simulink model "SimpleHumidifier_std"  (R2023b)
settings: Solver=ode4  StartTime=0.0  StopTime=10.0  FixedStep=1e-4  RelTol=1e-6
undefined symbols (not defined in the file): p_in_dry, p_in_wet, RH_in_dry, RH_in_wet, T_in_dry, T_in_wet, W_in_dry, W_in_wet, yO2_in_dry, yO2_in_wet
libraries: slpidlib x1
settings Model: Creator=KOTA-Z  LastModifiedBy=KOTA-Z

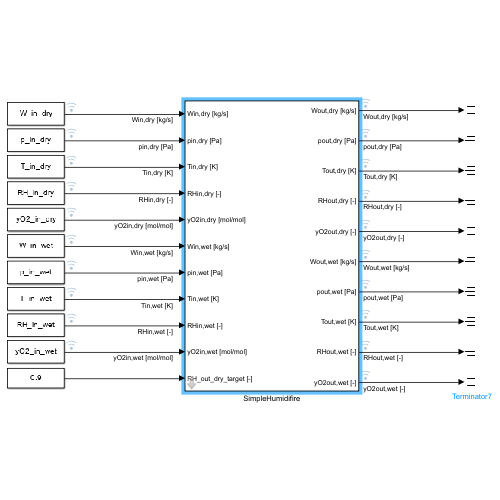
[thumbnail: Simulink's stored preview of the top-level diagram]
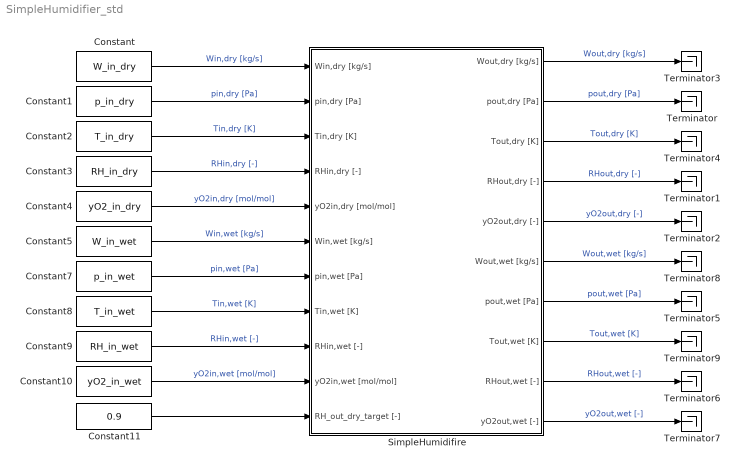
== system SimpleHumidifier_std ==
  Constant : Constant  Value=W_in_dry
  Constant1 : Constant  Value=p_in_dry
  Constant10 : Constant  Value=yO2_in_wet
  Constant11 : Constant  Value=0.9
  Constant2 : Constant  Value=T_in_dry
  Constant3 : Constant  Value=RH_in_dry
  Constant4 : Constant  Value=yO2_in_dry
  Constant5 : Constant  Value=W_in_wet
  Constant7 : Constant  Value=p_in_wet
  Constant8 : Constant  Value=T_in_wet
  Constant9 : Constant  Value=RH_in_wet
  SimpleHumidifire : Subsystem  mask(Simple FCstack){V_ca=1, A_ca=1, R_N2=1, R_O2=1, R_H2O=1, M_N2=1, M_O2=1, M_H2O=1}
      mask prompts: V_ca "Stack Volume (Cathode side) [m^3]"; A_ca "Stack Flow area (Cathode side) [m^2]"; R_N2 "Gas Constant N2 [J/kg/K]"; R_O2 "Gas Constant O2 [J/kg/K]"; R_H2O "Gas Constant H2O [J/kg/K]"; M_N2 "Molecular Weight N2 [kg/mol]"; M_O2 "Molecular Weight O2 [kg/mol]"; M_H2O "Molecular Weight H2O [kg/mol]"
      mask help: This block provides a simplified FCstack model. The reacted O2 and generated H2O in the stack are calculated based on lambda. Delay due to volume is considered and the pressure drop is approximated as the orifice law.
      mask DialogControl ParameterGroupVar Prompt: Geometric parameter
      mask DialogControl Container3 Prompt: Physical property
  Terminator{,1..9} (10 alike) : Terminator
  wires:
  Constant4/1 -> SimpleHumidifire/5(yO2in,dry [mol/mol])  "yO2in,dry [mol/mol]"
  Constant/1 -> SimpleHumidifire/1(Win,dry [kg/s])  "Win,dry [kg/s]"
  Constant3/1 -> SimpleHumidifire/4(RHin,dry [-])  "RHin,dry [-]"
  Constant1/1 -> SimpleHumidifire/2(pin,dry [Pa])  "pin,dry [Pa]"
  SimpleHumidifire/4(RHout,dry [-]) -> Terminator1/1  "RHout,dry [-]"
  SimpleHumidifire/1(Wout,dry [kg/s]) -> Terminator3/1  "Wout,dry [kg/s]"
  SimpleHumidifire/2(pout,dry [Pa]) -> Terminator/1  "pout,dry [Pa]"
  SimpleHumidifire/5(yO2out,dry [-]) -> Terminator2/1  "yO2out,dry [-]"
  Constant2/1 -> SimpleHumidifire/3(Tin,dry [K])  "Tin,dry [K]"
  SimpleHumidifire/3(Tout,dry [K]) -> Terminator4/1  "Tout,dry [K]"
  Constant8/1 -> SimpleHumidifire/8(Tin,wet [K])  "Tin,wet [K]"
  Constant5/1 -> SimpleHumidifire/6(Win,wet [kg/s])  "Win,wet [kg/s]"
  Constant7/1 -> SimpleHumidifire/7(pin,wet [Pa])  "pin,wet [Pa]"
  Constant9/1 -> SimpleHumidifire/9(RHin,wet [-])  "RHin,wet [-]"
  Constant10/1 -> SimpleHumidifire/10(yO2in,wet [mol/mol])  "yO2in,wet [mol/mol]"
  SimpleHumidifire/6(Wout,wet [kg/s]) -> Terminator8/1  "Wout,wet [kg/s]"
  SimpleHumidifire/10(yO2out,wet [-]) -> Terminator7/1  "yO2out,wet [-]"
  SimpleHumidifire/7(pout,wet [Pa]) -> Terminator5/1  "pout,wet [Pa]"
  SimpleHumidifire/9(RHout,wet [-]) -> Terminator6/1  "RHout,wet [-]"
  SimpleHumidifire/8(Tout,wet [K]) -> Terminator9/1  "Tout,wet [K]"
  Constant11/1 -> SimpleHumidifire/11(RH_out_dry_target [-])

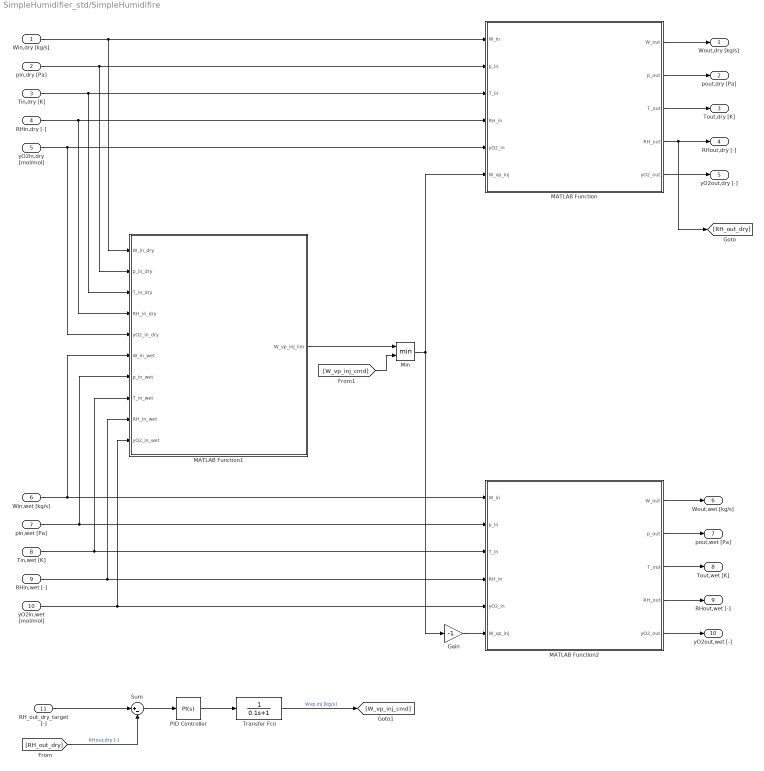
== system SimpleHumidifier_std/SimpleHumidifire ==
  Win,dry [kg/s] : Inport
  pin,dry [Pa] : Inport  Port=2
  Tin,dry [K] : Inport  Port=3
  RHin,dry [-] : Inport  Port=4
  yO2in,dry [mol/mol] : Inport  Port=5
  Win,wet [kg/s] : Inport  Port=6
  pin,wet [Pa] : Inport  Port=7
  Tin,wet [K] : Inport  Port=8
  RHin,wet [-] : Inport  Port=9
  yO2in,wet [mol/mol] : Inport  Port=10
  RH_out_dry_target [-] : Inport  Port=11
  Gain : Gain  Gain=-1
  MATLAB Function : MATLAB Function  TreatAsAtomicUnit=on
  MATLAB Function1 : MATLAB Function  TreatAsAtomicUnit=on
  MATLAB Function2 : MATLAB Function  TreatAsAtomicUnit=on
  Min : MinMax  Inputs=2
  PID Controller : slpidlib/PID Controller  Controller=PI  Form=Parallel  TimeDomain=Continuous-time  UseExternalTs=off  SampleTime=-1  IntegratorMethod=Forward Euler  FilterMethod=Forward Euler  ControllerParametersSource=internal  P=1  I=10  UseKiTs=off  D=0  N=100  UseFilter=on  TunerSelectOption=Transfer Function Based (PID Tuner App)  InitialConditionSource=internal  InitialConditionForIntegrator=0  InitialConditionForFilter=0  DifferentiatorICPrevScaledInput=0  ExternalReset=none  TrackingMode=off  Kt=1  LimitOutput=on  SatLimitsSource=internal  UpperSaturationLimit=1  LowerSaturationLimit=0  LinearizeAsGain=on  AntiWindupMode=back-calculation  Kb=1  LimitIntegrator=off  UpperIntegratorSaturationLimit=inf  LowerIntegratorSaturationLimit=-inf  POutMin=[]  POutMax=[]  IOutMin=[]  IOutMax=[]  DOutMin=[]  DOutMax=[]  NOutMin=[]  NOutMax=[]  SumOutMin=[]  SumOutMax=[]  SaturationOutMin=[]  SaturationOutMax=[]  PParamMin=[]  PParamMax=[]  IParamMin=[]  IParamMax=[]  DParamMin=[]  DParamMax=[]  NParamMin=[]  NParamMax=[]  KbParamMin=[]  KbParamMax=[]  KtParamMin=[]  KtParamMax=[]  KbOutMin=[]  KbOutMax=[]  KtOutMin=[]  KtOutMax=[]  IntegratorOutMin=[]  IntegratorOutMax=[]  FilterOutMin=[]  FilterOutMax=[]  SumI1OutMin=[]  SumI1OutMax=[]  SumI2OutMin=[]  SumI2OutMax=[]  SumI3OutMin=[]  SumI3OutMax=[]  SumI4OutMin=[]  SumI4OutMax=[]  SumDOutMin=[]  SumDOutMax=[]  DifferentiatorOutMin=[]  DifferentiatorOutMax=[]  FilterDiffOutCoefMin=[]  FilterDiffOutCoefMax=[]  ReciprocalOutMin=[]  ReciprocalOutMax=[]  SumDenOutMin=[]  SumDenOutMax=[]  SumNumOutMin=[]  SumNumOutMax=[]  DivideOutMin=[]  DivideOutMax=[]  UdiffTsProdOutMin=[]  UdiffTsProdOutMax=[]  NTsProdOutMin=[]  NTsProdOutMax=[]  UintegralTsProdOutMin=[]  UintegralTsProdOutMax=[]  UngainTsProdOutMin=[]  UngainTsProdOutMax=[]  ClampingZeroOutDataTypeStr=Inherit: Inherit via back propagation  ClampingZeroOutMin=[]  ClampingZeroOutMax=[]  FilterDenConstantOutDataTypeStr=Inherit: Inherit via back propagation  FilterDenConstantOutMin=[]  FilterDenConstantOutMax=[]  PCopyOutDataTypeStr=Inherit: Inherit via back propagation  PCopyOutMin=[]  PCopyOutMax=[]  NCopyOutDataTypeStr=Inherit: Inherit via back propagation  NCopyOutMin=[]  NCopyOutMax=[]  IntegratorContinuousStateAttributes=''  IntegratorStateMustResolveToSignalObject=off  IntegratorRTWStateStorageClass=Auto  FilterContinuousStateAttributes=''  FilterStateMustResolveToSignalObject=off  FilterRTWStateStorageClass=Auto  ParallelPVariant=InternalParameters  IdealPVariant=Disabled  IVariant=InternalParameters  DVariant=Disabled  IntegratorVariant=Continuous  SatVariant=Enabled  AWVariant=BackCalculation  PCopyVariant=Disabled  TRVariant=Disabled  FdbkBlocksVariant=Forward  IdealPFdbkVariant=Disabled  SatFdbkVariant=Disabled  DerivativeFilterVariant=Disabled  NVariant=Disabled  NCopyVariant=Disabled_SignalSpec  FilterICVariant=Disabled  IntegratorICVariant=InternalICs  ExternalResetVariant=Disabled  TRSumVariant=Passthrough  SumFdbkVariant=Disabled  SumVariant=Sum_PI  TsampFilterVariant=InternalTs  TsampNgainVariant=Passthrough  TsampIntegralVariant=Disabled_SignalSpec  ExternalSaturationOutDataTypeStr=Inherit: Same as second input
  Sum : Sum  Inputs=|+-
  Transfer Fcn : TransferFcn  Denominator=[0.1 1]
  Wout,dry [kg/s] : Outport
  pout,dry [Pa] : Outport  Port=2
  Tout,dry [K] : Outport  Port=3
  RHout,dry [-] : Outport  Port=4
  yO2out,dry [-] : Outport  Port=5
  Wout,wet [kg/s] : Outport  Port=6
  pout,wet [Pa] : Outport  Port=7
  Tout,wet [K] : Outport  Port=8
  RHout,wet [-] : Outport  Port=9
  yO2out,wet [-] : Outport  Port=10
  wires:
  MATLAB Function/5(yO2_out) -> yO2out,dry [-]/1
  MATLAB Function/2(p_out) -> pout,dry [Pa]/1
  MATLAB Function/1(W_out) -> Wout,dry [kg/s]/1
  MATLAB Function/4(RH_out) -> [RH_out_dry], RHout,dry [-]/1
  MATLAB Function/3(T_out) -> Tout,dry [K]/1
  pin,wet [Pa]/1 -> MATLAB Function1/7(p_in_wet), MATLAB Function2/2(p_in)
  Win,wet [kg/s]/1 -> MATLAB Function2/1(W_in), MATLAB Function1/6(W_in_wet)
  RHin,wet [-]/1 -> MATLAB Function1/9(RH_in_wet), MATLAB Function2/4(RH_in)
  RHin,dry [-]/1 -> MATLAB Function1/4(RH_in_dry), MATLAB Function/4(RH_in)
  pin,dry [Pa]/1 -> MATLAB Function1/2(p_in_dry), MATLAB Function/2(p_in)
  Tin,dry [K]/1 -> MATLAB Function1/3(T_in_dry), MATLAB Function/3(T_in)
  Win,dry [kg/s]/1 -> MATLAB Function1/1(W_in_dry), MATLAB Function/1(W_in)
  yO2in,wet [mol/mol]/1 -> MATLAB Function1/10(yO2_in_wet), MATLAB Function2/5(yO2_in)
  yO2in,dry [mol/mol]/1 -> MATLAB Function1/5(yO2_in_dry), MATLAB Function/5(yO2_in)
  Tin,wet [K]/1 -> MATLAB Function1/8(T_in_wet), MATLAB Function2/3(T_in)
  [W_vp_inj_cmd] -> Min/2
  MATLAB Function1/1(W_vp_inj_lim) -> Min/1
  Min/1 -> MATLAB Function/6(W_vp_inj), Gain/1
  Gain/1 -> MATLAB Function2/6(W_vp_inj)
  MATLAB Function2/1(W_out) -> Wout,wet [kg/s]/1
  MATLAB Function2/2(p_out) -> pout,wet [Pa]/1
  MATLAB Function2/3(T_out) -> Tout,wet [K]/1
  MATLAB Function2/4(RH_out) -> RHout,wet [-]/1
  MATLAB Function2/5(yO2_out) -> yO2out,wet [-]/1
  PID Controller/1 -> Transfer Fcn/1
  Transfer Fcn/1 -> [W_vp_inj_cmd]  "Wvp,inj [kg/s]"
  Sum/1 -> PID Controller/1
  RH_out_dry_target [-]/1 -> Sum/1
  [RH_out_dry] -> Sum/2  "RHout,dry [-]"

== matlab function SimpleHumidifier_std/SimpleHumidifire/MATLAB Function ==
  data: W_in input; W_out output; p_in input; T_in input; RH_in input; yO2_in input; W_vp_inj input; p_out output; T_out output; RH_out output; yO2_out output
%% 加湿／除湿計算（分圧ベース計算）
function [W_out, p_out, T_out, RH_out, yO2_out] = HM_std(W_in, p_in, T_in, RH_in, yO2_in, W_vp_inj)
    % 湿り空気の状態計算
    [W_O2_in, W_N2_in, W_vp_in, p_O2_in, p_N2_in, p_vp_in, M_in, R_in, cp_in, kap_in] = calc_MA_property(W_in, p_in, T_in, RH_in, yO2_in);

    % 水蒸気の注入
    W_vp_out = W_vp_in + W_vp_inj;  % [kg/s]

    % 出口流量計算
    W_O2_out = W_O2_in; % [kg/s]
    W_N2_out = W_N2_in; % [kg/s]
    W_out = W_O2_out + W_N2_out + W_vp_out; % [kg/s]

    % 出口圧計算
    p_O2_out = p_O2_in; % [Pa]
    p_N2_out = p_N2_in; % [Pa]
    if W_vp_out <= 0
        p_vp_out = 0;
    else
        p_vp_out = W_vp_out/W_vp_in * p_vp_in;  % [Pa]
    end
    p_out = p_O2_out + p_N2_out + p_vp_out;     % [Pa]

    % 温度は一定とする
    T_out = T_in;       % [K]

    % 相対湿度計算
    RH_out = p_vp_out/sat_vp_pressure(T_out);

    % 空気組成は一定とする
    yO2_out = yO2_in;   % [-]
end

%% 湿り空気の状態量計算
function [W_O2, W_N2, W_vp, p_O2, p_N2, p_vp, M, R, cp, kap] = calc_MA_property(W, p, T, RH, yO2)
    % 物理定数の定義
    % 分子量定義
    M_O2 = 32e-3;   % [kg/mol]
    M_N2 = 28e-3;   % [kg/mol]
    M_vp = 18e-3;   % [kg/mol]
    % 気体定数定義
    R0 = 8.31446261815324; % [J/K/mol]
    
    % 分圧計算
    p_vp_sat = sat_vp_pressure(T);
    p_vp = RH * p_vp_sat;
    p_DA = p - p_vp;
    p_O2 = yO2 * p_DA;
    p_N2 = p_DA - p_O2;
    
    % 湿り空気のモル分率計算
    x_O2 = p_O2/p;
    x_N2 = p_N2/p;
    x_vp = p_vp/p;

    % 湿り空気の分子量計算
    M = M_O2*x_O2 + M_N2*x_N2 + M_vp*x_vp;       % [kg/mol]

    % ガス定数計算
    R = R0/M;   % [J/K/kg]

    % 質量分率計算
    w_O2 = x_O2*M_O2 / M;
    w_N2 = x_N2*M_N2 / M;
    w_vp = x_vp*M_vp / M;

    % 各分子の定圧比熱の計算
    % 二原子分子
    cp_O2 = 7/2*R0 / M_O2;  % [J/K/kg]
    cp_N2 = 7/2*R0 / M_N2;  % [J/K/kg]
    % 水蒸気
    cp_vp = 4*R0 / M_vp;    % [J/K/kg]

    % 混合気体の定圧比熱
    cp = cp_O2*w_O2 + cp_N2*w_N2 + cp_vp*w_vp;  % [J/K/kg]

    % 混合気体の比熱比
    kap = cp/(cp-R);

    % 各分子の質量流量
    W_O2 = W * w_O2;    % [kg/s]
    W_N2 = W * w_N2;    % [kg/s]
    W_vp = W * w_vp;    % [kg/s]
end

%% Calculate saturated vapor pressure [Pa]
function psat = sat_vp_pressure(Ts)
    P_CONVERT = 0.001;
    C1 = -5.6745359e3;
    C2 = 6.3925247;
    C3 = -9.6778430e-3;
    C4 = 6.2215701e-7;
    C5 = 2.0747825e-9;
    C6 = -9.4840240e-13;
    C7 = 4.1635019;
    N1 = 0.11670521452767e4;
    N2 = -0.72421316703206e6;
    N3 = -0.17073846940092e2;
    N4 = 0.12020824702470e5;
    N5 = -0.32325550322333e7;
    N6 = 0.14915108613530e2;
    N7 = -0.4823265731591e4;
    N8 = 0.40511340542057e6;
    N9 = -0.23855557567849e0;
    N10 = 0.65017534844798e3;
    
    if Ts < 273.15+0.01
        % -100~0.01C//三重点を計算以下は wexler-hyland のシミュレーションプログラム式
        psat = exp(C1 / Ts + C2 + C3 * Ts + C4 * Ts^2 + C5 * Ts^3 + C6 * Ts^4 + C7 * log(Ts)) * P_CONVERT;
    else
        %　~647.096K//臨界温度まで一定とするは IAPWS-IF97 実用国際状態式
        alpha = Ts + N9 / (Ts - N10);
        a2 = alpha * alpha;
        A = a2 + N1 * alpha + N2;
        B = N3 * a2 + N4 * alpha + N5;
        C = N6 * a2 + N7 * alpha + N8;
        psat = (2 * C / (-B + (B * B - 4 * A * C)^0.5))^4 / P_CONVERT;
    end 
    psat = psat*1000; %kPa to Pa
end

== matlab function SimpleHumidifier_std/SimpleHumidifire/MATLAB Function1 ==
  data: W_in_dry input; W_vp_inj_lim output; p_in_dry input; T_in_dry input; RH_in_dry input; yO2_in_dry input; W_in_wet input; p_in_wet input; T_in_wet input; RH_in_wet input; yO2_in_wet input
%% 水交換量のリミット計算
function W_vp_inj_lim = calc_W_vp_inj_lim(W_in_dry, p_in_dry, T_in_dry, RH_in_dry, yO2_in_dry,W_in_wet, p_in_wet, T_in_wet, RH_in_wet, yO2_in_wet)
    % 物理定数の定義
    % 分子量定義
    % M_O2 = 32e-3;   % [kg/mol]
    % M_N2 = 28e-3;   % [kg/mol]
    M_vp = 18e-3;   % [kg/mol]

    % 湿り空気の分圧計算
    % DRY側
    [W_O2_in_dry, W_N2_in_dry, W_vp_in_dry, p_O2_in_dry, p_N2_in_dry, p_vp_in_dry, M_in_dry, R_in_dry, cp_in_dry, kap_in_dry] = calc_MA_property(W_in_dry, p_in_dry, T_in_dry, RH_in_dry, yO2_in_dry);
    % WET側
    [W_O2_in_wet, W_N2_in_wet, W_vp_in_wet, p_O2_in_wet, p_N2_in_wet, p_vp_in_wet, M_in_wet, R_in_wet, cp_in_wet, kap_in_wet] = calc_MA_property(W_in_wet, p_in_wet, T_in_wet, RH_in_wet, yO2_in_wet);

    % DRY側リミット
    % RH=1の時の水蒸気流量
    W_vp_RH1 = sat_vp_pressure(T_in_dry)/p_in_dry * M_vp/M_in_dry * W_in_dry;       % 湿り空気ベース計算
    % W_vp_RH1 = sat_vp_pressure(T_in_dry)/p_O2_in_dry * M_vp/M_O2 * W_O2_in_dry;   % 酸素ベース計算
    % W_vp_RH1 = sat_vp_pressure(T_in_dry)/(p_O2_in_dry+p_N2_in_dry) * M_vp/(yO2_in_dry*M_O2+(1-yO2_in_dry)*M_N2) * (W_O2_in_dry+W_N2_in_dry); % 乾燥空気ベース計算
    % リミット交換量
    W_vp_inj_lim_dry =  W_vp_RH1 - W_vp_in_dry;

    % WET側リミット
    W_vp_inj_lim_wet =  W_vp_in_wet - 0;

    % 小さいほうがリミットとなる
    W_vp_inj_lim = min(W_vp_inj_lim_dry, W_vp_inj_lim_wet);
end

%% 湿り空気の状態量計算
function [W_O2, W_N2, W_vp, p_O2, p_N2, p_vp, M, R, cp, kap] = calc_MA_property(W, p, T, RH, yO2)
    % 物理定数の定義
    % 分子量定義
    M_O2 = 32e-3;   % [kg/mol]
    M_N2 = 28e-3;   % [kg/mol]
    M_vp = 18e-3;   % [kg/mol]
    % 気体定数定義
    R0 = 8.31446261815324; % [J/K/mol]
    
    % 分圧計算
    p_vp_sat = sat_vp_pressure(T);
    p_vp = RH * p_vp_sat;
    p_DA = p - p_vp;
    p_O2 = yO2 * p_DA;
    p_N2 = p_DA - p_O2;
    
    % 湿り空気のモル分率計算
    x_O2 = p_O2/p;
    x_N2 = p_N2/p;
    x_vp = p_vp/p;

    % 湿り空気の分子量計算
    M = M_O2*x_O2 + M_N2*x_N2 + M_vp*x_vp;       % [kg/mol]

    % ガス定数計算
    R = R0/M;   % [J/K/kg]

    % 質量分率計算
    w_O2 = x_O2*M_O2 / M;
    w_N2 = x_N2*M_N2 / M;
    w_vp = x_vp*M_vp / M;

    % 各分子の定圧比熱の計算
    % 二原子分子
    cp_O2 = 7/2*R0 / M_O2;  % [J/K/kg]
    cp_N2 = 7/2*R0 / M_N2;  % [J/K/kg]
    % 水蒸気
    cp_vp = 4*R0 / M_vp;    % [J/K/kg]

    % 混合気体の定圧比熱
    cp = cp_O2*w_O2 + cp_N2*w_N2 + cp_vp*w_vp;  % [J/K/kg]

    % 混合気体の比熱比
    kap = cp/(cp-R);

    % 各分子の質量流量
    W_O2 = W * w_O2;    % [kg/s]
    W_N2 = W * w_N2;    % [kg/s]
    W_vp = W * w_vp;    % [kg/s]
end

%% Calculate saturated vapor pressure [Pa]
function psat = sat_vp_pressure(Ts)
    P_CONVERT = 0.001;
    C1 = -5.6745359e3;
    C2 = 6.3925247;
    C3 = -9.6778430e-3;
    C4 = 6.2215701e-7;
    C5 = 2.0747825e-9;
    C6 = -9.4840240e-13;
    C7 = 4.1635019;
    N1 = 0.11670521452767e4;
    N2 = -0.72421316703206e6;
    N3 = -0.17073846940092e2;
    N4 = 0.12020824702470e5;
    N5 = -0.32325550322333e7;
    N6 = 0.14915108613530e2;
    N7 = -0.4823265731591e4;
    N8 = 0.40511340542057e6;
    N9 = -0.23855557567849e0;
    N10 = 0.65017534844798e3;
    
    if Ts < 273.15+0.01
        % -100~0.01C//三重点を計算以下は wexler-hyland のシミュレーションプログラム式
        psat = exp(C1 / Ts + C2 + C3 * Ts + C4 * Ts^2 + C5 * Ts^3 + C6 * Ts^4 + C7 * log(Ts)) * P_CONVERT;
    else
        %　~647.096K//臨界温度まで一定とするは IAPWS-IF97 実用国際状態式
        alpha = Ts + N9 / (Ts - N10);
        a2 = alpha * alpha;
        A = a2 + N1 * alpha + N2;
        B = N3 * a2 + N4 * alpha + N5;
        C = N6 * a2 + N7 * alpha + N8;
        psat = (2 * C / (-B + (B * B - 4 * A * C)^0.5))^4 / P_CONVERT;
    end 
    psat = psat*1000; %kPa to Pa
end

== matlab function SimpleHumidifier_std/SimpleHumidifire/MATLAB Function2 ==
  data: W_in input; W_out output; p_in input; T_in input; RH_in input; yO2_in input; W_vp_inj input; p_out output; T_out output; RH_out output; yO2_out output
%% 加湿／除湿計算（分圧ベース計算）
function [W_out, p_out, T_out, RH_out, yO2_out] = HM_std(W_in, p_in, T_in, RH_in, yO2_in, W_vp_inj)
    % 湿り空気の状態計算
    [W_O2_in, W_N2_in, W_vp_in, p_O2_in, p_N2_in, p_vp_in, M_in, R_in, cp_in, kap_in] = calc_MA_property(W_in, p_in, T_in, RH_in, yO2_in);

    % 水蒸気の注入
    W_vp_out = W_vp_in + W_vp_inj;  % [kg/s]

    % 出口流量計算
    W_O2_out = W_O2_in; % [kg/s]
    W_N2_out = W_N2_in; % [kg/s]
    W_out = W_O2_out + W_N2_out + W_vp_out; % [kg/s]

    % 出口圧計算
    p_O2_out = p_O2_in; % [Pa]
    p_N2_out = p_N2_in; % [Pa]
    if W_vp_out <= 0
        p_vp_out = 0;
    else
        p_vp_out = W_vp_out/W_vp_in * p_vp_in;  % [Pa]
    end
    p_out = p_O2_out + p_N2_out + p_vp_out;     % [Pa]

    % 温度は一定とする
    T_out = T_in;       % [K]

    % 相対湿度計算
    RH_out = p_vp_out/sat_vp_pressure(T_out);

    % 空気組成は一定とする
    yO2_out = yO2_in;   % [-]
end

%% 湿り空気の状態量計算
function [W_O2, W_N2, W_vp, p_O2, p_N2, p_vp, M, R, cp, kap] = calc_MA_property(W, p, T, RH, yO2)
    % 物理定数の定義
    % 分子量定義
    M_O2 = 32e-3;   % [kg/mol]
    M_N2 = 28e-3;   % [kg/mol]
    M_vp = 18e-3;   % [kg/mol]
    % 気体定数定義
    R0 = 8.31446261815324; % [J/K/mol]
    
    % 分圧計算
    p_vp_sat = sat_vp_pressure(T);
    p_vp = RH * p_vp_sat;
    p_DA = p - p_vp;
    p_O2 = yO2 * p_DA;
    p_N2 = p_DA - p_O2;
    
    % 湿り空気のモル分率計算
    x_O2 = p_O2/p;
    x_N2 = p_N2/p;
    x_vp = p_vp/p;

    % 湿り空気の分子量計算
    M = M_O2*x_O2 + M_N2*x_N2 + M_vp*x_vp;       % [kg/mol]

    % ガス定数計算
    R = R0/M;   % [J/K/kg]

    % 質量分率計算
    w_O2 = x_O2*M_O2 / M;
    w_N2 = x_N2*M_N2 / M;
    w_vp = x_vp*M_vp / M;

    % 各分子の定圧比熱の計算
    % 二原子分子
    cp_O2 = 7/2*R0 / M_O2;  % [J/K/kg]
    cp_N2 = 7/2*R0 / M_N2;  % [J/K/kg]
    % 水蒸気
    cp_vp = 4*R0 / M_vp;    % [J/K/kg]

    % 混合気体の定圧比熱
    cp = cp_O2*w_O2 + cp_N2*w_N2 + cp_vp*w_vp;  % [J/K/kg]

    % 混合気体の比熱比
    kap = cp/(cp-R);

    % 各分子の質量流量
    W_O2 = W * w_O2;    % [kg/s]
    W_N2 = W * w_N2;    % [kg/s]
    W_vp = W * w_vp;    % [kg/s]
end

%% Calculate saturated vapor pressure [Pa]
function psat = sat_vp_pressure(Ts)
    P_CONVERT = 0.001;
    C1 = -5.6745359e3;
    C2 = 6.3925247;
    C3 = -9.6778430e-3;
    C4 = 6.2215701e-7;
    C5 = 2.0747825e-9;
    C6 = -9.4840240e-13;
    C7 = 4.1635019;
    N1 = 0.11670521452767e4;
    N2 = -0.72421316703206e6;
    N3 = -0.17073846940092e2;
    N4 = 0.12020824702470e5;
    N5 = -0.32325550322333e7;
    N6 = 0.14915108613530e2;
    N7 = -0.4823265731591e4;
    N8 = 0.40511340542057e6;
    N9 = -0.23855557567849e0;
    N10 = 0.65017534844798e3;
    
    if Ts < 273.15+0.01
        % -100~0.01C//三重点を計算以下は wexler-hyland のシミュレーションプログラム式
        psat = exp(C1 / Ts + C2 + C3 * Ts + C4 * Ts^2 + C5 * Ts^3 + C6 * Ts^4 + C7 * log(Ts)) * P_CONVERT;
    else
        %　~647.096K//臨界温度まで一定とするは IAPWS-IF97 実用国際状態式
        alpha = Ts + N9 / (Ts - N10);
        a2 = alpha * alpha;
        A = a2 + N1 * alpha + N2;
        B = N3 * a2 + N4 * alpha + N5;
        C = N6 * a2 + N7 * alpha + N8;
        psat = (2 * C / (-B + (B * B - 4 * A * C)^0.5))^4 / P_CONVERT;
    end 
    psat = psat*1000; %kPa to Pa
end
